simulink model "array_2x2"  (R2025b)
settings: Solver=VariableStepAuto  StartTime=0.0  StopTime=10.0  RelTol=1e-3
model workspace (MAT data in the model file):
  FL = 10
  Sig = Simulink.Signal
  Sig.Dimensions = -1
  Sig.DimensionsMode = 'auto'
  Sig.Complexity = 'auto'
  Sig.SampleTime = -1
  Sig.SamplingMode = 'auto'
  Sig.DataType = 'auto'
  WL = 10
settings Model: Creator=Andrei  LastModifiedBy=Andrei

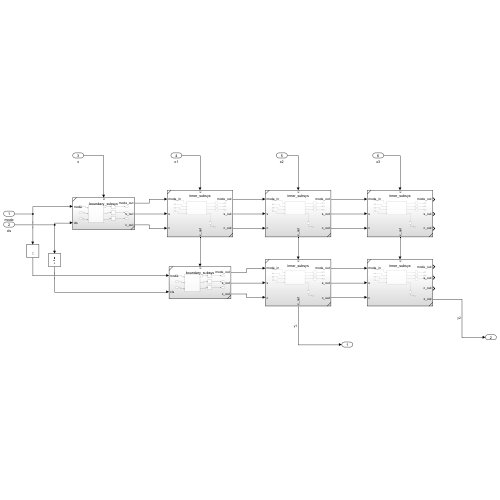
[thumbnail: Simulink's stored preview of the top-level diagram]
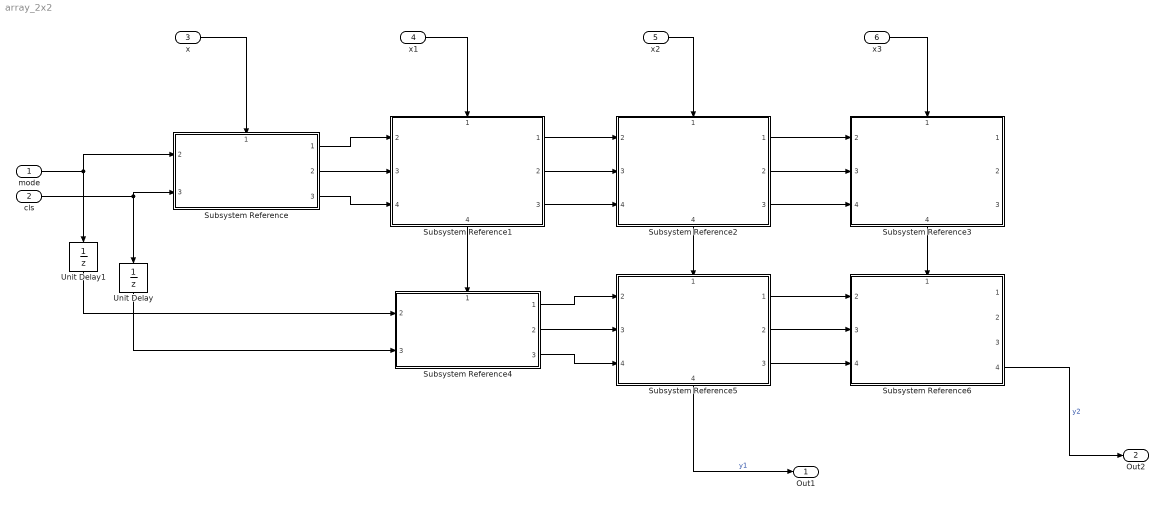
== system array_2x2 ==
  mode : Inport
  cls : Inport  Port=2
  x : Inport  Port=3  OutDataTypeStr=fixdt(1,WL,FL)
  x1 : Inport  Port=4  OutDataTypeStr=fixdt(1,WL,FL)
  x2 : Inport  Port=5  OutDataTypeStr=fixdt(1,WL,FL)
  x3 : Inport  Port=6  OutDataTypeStr=fixdt(1,WL,FL)
  Subsystem Reference : Subsystem  ReferencedSubsystem=boundary_subsys
      settings: PortSchema="{\"entries\":[{\"content\":{\"sides\":[{\"content\":{\"connectorIds\":[\"In2\",\"In3\"]},\"type\":\"ConnectorPlacement.EquallySpacedRectSide\",\"uuid\":\"92a343e4-4510-496d-8069-d6a4c9d6bf12\"},{\"content\":{\"connectorIds\":[\"Out1\",\"Out2\",\"Out3\"],\"side\":\"RIGHT\"},\"type\":\"ConnectorPlacement.EquallySpacedRectSide\",\"uuid\":\"d7c10f84-3430-4177-9926-c1fb8da23e20\"},{\"content\":{\"connectorIds\":[\"In1\"],\"side\":\"TOP\"},\"type\":\"ConnectorPlacement.EquallySpacedRectSide\",\"uuid\":\"976898b3-1521-4361-83a1-553737f64a39\"}]},\"type\":\"ConnectorPlacement.EquallySpacedConnector\",\"uuid\":\"3ce70afe-f04a-487e-8641-2fe6ce8ccb50\"}],\"packageUris\":[\"http://schema.mathworks.com/mf0/Connector/R2020b\"],\"version\":\"1.0\"}"
  Subsystem Reference{1..3,5..6} (5 alike) : Subsystem  ReferencedSubsystem=inner_subsys
      Subsystem Reference1 settings: PortSchema="{\"entries\":[{\"content\":{\"sides\":[{\"content\":{\"connectorIds\":[\"In2\",\"In3\",\"In4\"]},\"type\":\"ConnectorPlacement.EquallySpacedRectSide\",\"uuid\":\"dbc71003-5ddd-4d69-8235-df2a7eac87fb\"},{\"content\":{\"connectorIds\":[\"Out1\",\"Out2\",\"Out3\"],\"side\":\"RIGHT\"},\"type\":\"ConnectorPlacement.EquallySpacedRectSide\",\"uuid\":\"acfb1494-fa6e-460c-affc-491b01631d29\"},{\"content\":{\"connectorIds\":[\"In1\"],\"side\":\"TOP\"},\"type\":\"ConnectorPlacement.EquallySpacedRectSide\",\"uuid\":\"9df206bd-5e7b-487b-8848-9d6785089e3f\"},{\"content\":{\"connectorIds\":[\"Out4\"],\"side\":\"BOTTOM\"},\"type\":\"ConnectorPlacement.EquallySpacedRectSide\",\"uuid\":\"a65c56a2-914f-4631-8a73-1db54343e3c8\"}]},\"type\":\"ConnectorPlacement.EquallySpacedConnector\",\"uuid\":\"2594815e-50bc-4ec3-bffd-73d6907b23c8\"}],\"packageUris\":[\"http://schema.mathworks.com/mf0/Connector/R2020b\"],\"version\":\"1.0\"}"
      Subsystem Reference2 settings: PortSchema="{\"entries\":[{\"content\":{\"sides\":[{\"content\":{\"connectorIds\":[\"In2\",\"In3\",\"In4\"]},\"type\":\"ConnectorPlacement.EquallySpacedRectSide\",\"uuid\":\"dbc71003-5ddd-4d69-8235-df2a7eac87fb\"},{\"content\":{\"connectorIds\":[\"Out1\",\"Out2\",\"Out3\"],\"side\":\"RIGHT\"},\"type\":\"ConnectorPlacement.EquallySpacedRectSide\",\"uuid\":\"acfb1494-fa6e-460c-affc-491b01631d29\"},{\"content\":{\"connectorIds\":[\"In1\"],\"side\":\"TOP\"},\"type\":\"ConnectorPlacement.EquallySpacedRectSide\",\"uuid\":\"9df206bd-5e7b-487b-8848-9d6785089e3f\"},{\"content\":{\"connectorIds\":[\"Out4\"],\"side\":\"BOTTOM\"},\"type\":\"ConnectorPlacement.EquallySpacedRectSide\",\"uuid\":\"8966e87e-b0a8-4cc4-bc92-71ad54fbd042\"}]},\"type\":\"ConnectorPlacement.EquallySpacedConnector\",\"uuid\":\"2594815e-50bc-4ec3-bffd-73d6907b23c8\"}],\"packageUris\":[\"http://schema.mathworks.com/mf0/Connector/R2020b\"],\"version\":\"1.0\"}"
      Subsystem Reference3 settings: PortSchema="{\"entries\":[{\"content\":{\"sides\":[{\"content\":{\"connectorIds\":[\"In2\",\"In3\",\"In4\"]},\"type\":\"ConnectorPlacement.EquallySpacedRectSide\",\"uuid\":\"dbc71003-5ddd-4d69-8235-df2a7eac87fb\"},{\"content\":{\"connectorIds\":[\"Out1\",\"Out2\",\"Out3\"],\"side\":\"RIGHT\"},\"type\":\"ConnectorPlacement.EquallySpacedRectSide\",\"uuid\":\"acfb1494-fa6e-460c-affc-491b01631d29\"},{\"content\":{\"connectorIds\":[\"In1\"],\"side\":\"TOP\"},\"type\":\"ConnectorPlacement.EquallySpacedRectSide\",\"uuid\":\"9df206bd-5e7b-487b-8848-9d6785089e3f\"},{\"content\":{\"connectorIds\":[\"Out4\"],\"side\":\"BOTTOM\"},\"type\":\"ConnectorPlacement.EquallySpacedRectSide\",\"uuid\":\"2e8e6e29-b6f8-437f-8718-04defcb9d1be\"}]},\"type\":\"ConnectorPlacement.EquallySpacedConnector\",\"uuid\":\"2594815e-50bc-4ec3-bffd-73d6907b23c8\"}],\"packageUris\":[\"http://schema.mathworks.com/mf0/Connector/R2020b\"],\"version\":\"1.0\"}"
      Subsystem Reference5 settings: PortSchema="{\"entries\":[{\"content\":{\"sides\":[{\"content\":{\"connectorIds\":[\"In2\",\"In3\",\"In4\"]},\"type\":\"ConnectorPlacement.EquallySpacedRectSide\",\"uuid\":\"dbc71003-5ddd-4d69-8235-df2a7eac87fb\"},{\"content\":{\"connectorIds\":[\"Out1\",\"Out2\",\"Out3\"],\"side\":\"RIGHT\"},\"type\":\"ConnectorPlacement.EquallySpacedRectSide\",\"uuid\":\"acfb1494-fa6e-460c-affc-491b01631d29\"},{\"content\":{\"connectorIds\":[\"In1\"],\"side\":\"TOP\"},\"type\":\"ConnectorPlacement.EquallySpacedRectSide\",\"uuid\":\"9df206bd-5e7b-487b-8848-9d6785089e3f\"},{\"content\":{\"connectorIds\":[\"Out4\"],\"side\":\"BOTTOM\"},\"type\":\"ConnectorPlacement.EquallySpacedRectSide\",\"uuid\":\"f5ac06d2-d4e5-4499-bb33-6140b0a1c1fa\"}]},\"type\":\"ConnectorPlacement.EquallySpacedConnector\",\"uuid\":\"2594815e-50bc-4ec3-bffd-73d6907b23c8\"}],\"packageUris\":[\"http://schema.mathworks.com/mf0/Connector/R2020b\"],\"version\":\"1.0\"}"
      Subsystem Reference6 settings: PortSchema="{\"entries\":[{\"content\":{\"sides\":[{\"content\":{\"connectorIds\":[\"In2\",\"In3\",\"In4\"]},\"type\":\"ConnectorPlacement.EquallySpacedRectSide\",\"uuid\":\"dbc71003-5ddd-4d69-8235-df2a7eac87fb\"},{\"content\":{\"connectorIds\":[\"Out1\",\"Out2\",\"Out3\",\"Out4\"],\"side\":\"RIGHT\"},\"type\":\"ConnectorPlacement.EquallySpacedRectSide\",\"uuid\":\"acfb1494-fa6e-460c-affc-491b01631d29\"},{\"content\":{\"connectorIds\":[\"In1\"],\"side\":\"TOP\"},\"type\":\"ConnectorPlacement.EquallySpacedRectSide\",\"uuid\":\"9df206bd-5e7b-487b-8848-9d6785089e3f\"}]},\"type\":\"ConnectorPlacement.EquallySpacedConnector\",\"uuid\":\"2594815e-50bc-4ec3-bffd-73d6907b23c8\"}],\"packageUris\":[\"http://schema.mathworks.com/mf0/Connector/R2020b\"],\"version\":\"1.0\"}"
  Subsystem Reference4 : Subsystem  ReferencedSubsystem=boundary_subsys
      settings: PortSchema="{\"entries\":[{\"content\":{\"sides\":[{\"content\":{\"connectorIds\":[\"In2\",\"In3\"]},\"type\":\"ConnectorPlacement.EquallySpacedRectSide\",\"uuid\":\"92a343e4-4510-496d-8069-d6a4c9d6bf12\"},{\"content\":{\"connectorIds\":[\"Out1\",\"Out2\",\"Out3\"],\"side\":\"RIGHT\"},\"type\":\"ConnectorPlacement.EquallySpacedRectSide\",\"uuid\":\"d7c10f84-3430-4177-9926-c1fb8da23e20\"},{\"content\":{\"connectorIds\":[\"In1\"],\"side\":\"TOP\"},\"type\":\"ConnectorPlacement.EquallySpacedRectSide\",\"uuid\":\"976898b3-1521-4361-83a1-553737f64a39\"}]},\"type\":\"ConnectorPlacement.EquallySpacedConnector\",\"uuid\":\"3ce70afe-f04a-487e-8641-2fe6ce8ccb50\"}],\"packageUris\":[\"http://schema.mathworks.com/mf0/Connector/R2020b\"],\"version\":\"1.0\"}"
  Unit Delay : UnitDelay  SampleTime=-1  HasFrameUpgradeWarning=on
  Unit Delay1 : UnitDelay  SampleTime=-1  HasFrameUpgradeWarning=on
  Out1 : Outport
  Out2 : Outport  Port=2
  wires:
  Subsystem Reference/1 -> Subsystem Reference1/2
  Subsystem Reference/2 -> Subsystem Reference1/3
  Subsystem Reference/3 -> Subsystem Reference1/4
  Subsystem Reference1/1 -> Subsystem Reference2/2
  Subsystem Reference1/2 -> Subsystem Reference2/3
  Subsystem Reference2/1 -> Subsystem Reference3/2
  Subsystem Reference2/2 -> Subsystem Reference3/3
  Subsystem Reference2/3 -> Subsystem Reference3/4
  Subsystem Reference1/4 -> Subsystem Reference4/1
  Subsystem Reference4/1 -> Subsystem Reference5/2
  Subsystem Reference4/2 -> Subsystem Reference5/3
  Subsystem Reference4/3 -> Subsystem Reference5/4
  Subsystem Reference2/4 -> Subsystem Reference5/1
  Subsystem Reference5/1 -> Subsystem Reference6/2
  Subsystem Reference5/2 -> Subsystem Reference6/3
  Subsystem Reference5/3 -> Subsystem Reference6/4
  Subsystem Reference3/4 -> Subsystem Reference6/1
  Subsystem Reference1/3 -> Subsystem Reference2/4
  cls/1 -> Unit Delay/1, Subsystem Reference/3
  mode/1 -> Unit Delay1/1, Subsystem Reference/2
  Subsystem Reference5/4 -> Out1/1  "y1"
  Subsystem Reference6/4 -> Out2/1  "y2"
  Unit Delay/1 -> Subsystem Reference4/3
  Unit Delay1/1 -> Subsystem Reference4/2
  x/1 -> Subsystem Reference/1
  x1/1 -> Subsystem Reference1/1
  x2/1 -> Subsystem Reference2/1
  x3/1 -> Subsystem Reference3/1
